simulink model "iso_force_production"  (R2015a)
settings: Solver=ode4  SolverMode=MultiTasking  StartTime=0.0  StopTime=inf  FixedStep=BKIN_STEP_TIME  RelTol=1e-3
StartFcn:
  |  warndlg('Dexterit-E models cannot run under simulation. Please compile your model and run it from within Dexterit-E.');set_param(bdroot,'SimulationCommand','stop')
model workspace (MAT data in the model file):
  BKIN_STEP_TIME = 0.00025
  col_x = 1
  col_y = 2
  VRAD = 3
  COLOR = 4
  TARGET_COL = 1
  BKIN_KINEMATIC_FRAME_SIZE = 400
  E_NO_EVENT = 0
  K_START_TGT = 1
  INIT_DUR = 4
  TP_ITI = 8
  K_JOINT_ASSESSED = 2
  TEXT1 = 5
  TEXT2 = 6
  HEIGHT = 7
  STROKE_WIDTH = 8
  GOAL_F_PCT = 2
  DO_FDBK = 7
  MAX_MOVE_TIME = 6
  FORCE_HOLD_TIME = 5
  MIN_FORCE = 3
  E_TEST_MVC = 1
  E_HOLD_MVC = 3
  E_EOT = 10
  E_FORCE_TRIAL = 2
  E_HOLD_FORCE = 4
libraries: Video x4, General x3, KINARM_loads x2, slrtlib x2, KINARM_IO x1, simulink x1
CloseFcn:
  | rtwprivate ssgencode ModelCloseRequest b2lab2d
settings Model: ModifiedComment=chris -- Wed Feb 16 09:18:30 2005 -- Version 1.1384  ExtModeArmWhenConnect=off  ExtModeLogAll=off  LastModifiedBy=Aaron
settings SolverCC: EnableConcurrentExecution=on  AutoInsertRateTranBlk=on
settings DataIOCC: LimitDataPoints=off  SignalLoggingSaveFormat=ModelDataLogs  SaveOutput=off  SaveTime=off  SignalLoggingName=sigsOut
settings OptimizationCC: BlockReduction=off  BooleanDataType=off  OptimizeBlockIOStorage=off  BufferReuse=off  GlobalBufferReuse=off  ExpressionFolding=off  ExpressionDepthLimit=2147483647  LocalBlockOutputs=off  InitFltsAndDblsToZero=on
settings DebuggingCC: SaveWithParameterizedLinksMsg=none  UnderspecifiedInitializationDetection=Classic  MergeDetectMultiDrivingBlocksExec=none  SignalResolutionControl=TryResolveAllWithWarning  MultiTaskDSMMsg=warning  FcnCallInpInsideContextMsg=UseLocalSettings  StateNameClashWarn=warning  StrictBusMsg=ErrorOnBusTreatedAsVector
settings HardwareCC: ProdIntDivRoundTo=Zero  ProdEndianess=LittleEndian  ProdLongLongMode=on  ProdHWDeviceType=Generic->32-bit x86 compatible  TargetHWDeviceType=32-bit Generic
settings SFSimCC: SimParseCustomCode=off
settings RTWCC: SystemTargetFile=slrt.tlc  TemplateMakefile=slrt_default_tmf  Description=Simulink Real-Time  RTWCompilerOptimization=on
settings CodeAppCC: MaxIdLength=63
settings SimulinkRealTimeCC: TargetFcnLib=ansi_tfl_tmw.mat  GeneratePreprocessorConditionals=Disable all  xPCisDownloadable=off

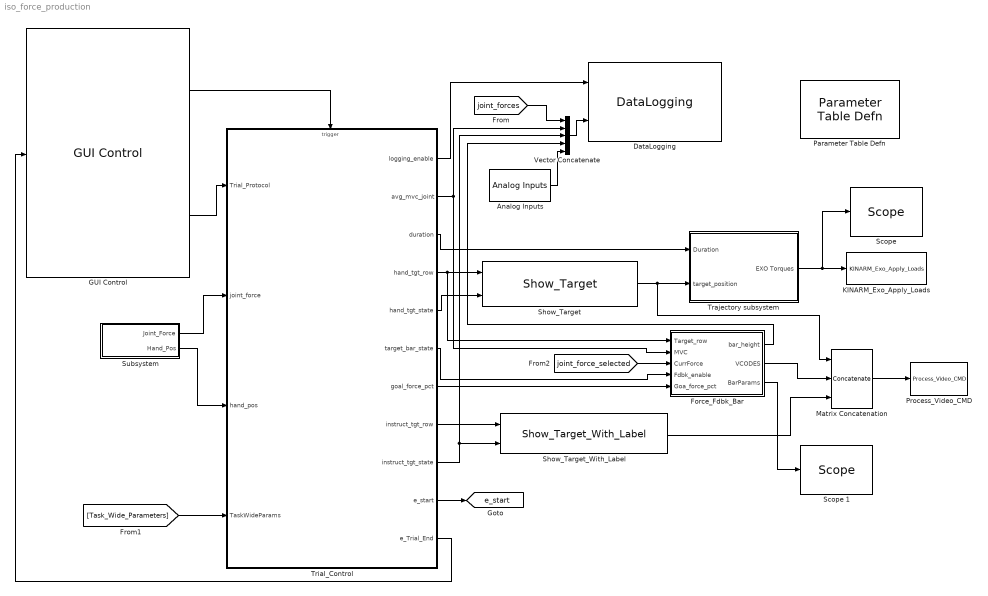
== system iso_force_production ==
  Analog Inputs : KINARM_IO/Analog Inputs  channel=[1]  range=[5]  coupling=[0]  scantime6071e=1.28e-5  scantime6229=5e-6  sampletime=0.001  slot=-1  oscantime6071e=0
  DataLogging : General/DataLogging  log_event_codes=off  log_analog_inputs=on  show_time_remaining=off  ecat_include=on
      link override Poll KINARM/EPTorqueCMD: GotoTag=KINARMEPTorqueCMD
      link override Poll KINARM/TorqueCMD: GotoTag=KINARMTorqueCMD
  Force_Fdbk_Bar : Subsystem
  GUI Control : General/GUI Control  task_version=1.0  show_repeat_trial_flag=off  use_custom_tp=off  target_type_str=Circle  Target_Type=1  XYcols=[1 2]  Vcols=3  Lcols=4  indices_padding=[0 0 0 0;0 0 0 0]  target_table_rows=64  load_table_rows=20  tp_table_rows=100
  KINARM_Exo_Apply_Loads : KINARM_loads/KINARM_Exo_Apply_Loads  up_duration=1000  down_duration=1000  max_torque=1  limit_motors=off
  Matrix Concatenation : Concatenate  NumInputs=3  Mode=Multidimensional array
  Parameter Table Defn : General/Parameter Table Defn  ShowInLibBrowser=0
  Process_Video_CMD : Video/Process_Video_CMD  video_delay=0
  "Scope " : slrtlib/Displays and Logging/Scope   scopeno=1  scopetype=Target  autostart=on  viewmode=Numerical  formatstr='%15.6f'  grid=on  ylimits=[0,0]  nosamples=250  noprepostsamples=0  interleave=1  triggermode=FreeRun  triggersignal=1  trigsignalfromport=off  triggerlevel=0.0  triggerslope=Either  triggerscope=1  triggersample=0  filename=data.dat  mode=Lazy  writesize=512  autorestart=off  dynamicfilemode=off  maxwritefilesize=512*1024^2
  Scope 1 : slrtlib/Displays and Logging/Scope   scopeno=2  scopetype=Target  autostart=on  viewmode=Numerical  formatstr='%15.6f'  grid=on  ylimits=[0,0]  nosamples=250  noprepostsamples=0  interleave=1  triggermode=FreeRun  triggersignal=1  trigsignalfromport=off  triggerlevel=0.0  triggerslope=Either  triggerscope=1  triggersample=0  filename=data.dat  mode=Lazy  writesize=512  autorestart=off  dynamicfilemode=off  maxwritefilesize=512*1024^2
  Show_Target : Video/Show_Target  target_type=Circle  num_states=1  attribcol1=[COLOR 0 0 VRAD]  attribcol2=[0 0 0 0]  attribcol3=[0 0 0 0]  attribcol4=[0 0 0 0]  attribcol5=[0 0 0 0]  stateindices_padding=[0 0 0 0 0 0 0;0 0 0 0 0 0 0;0 0 0 0 0 0 0;0 0 0 0 0 0 0;0 0 0 0 0 0 0]  source=dialog  opacity=100  target_display=Both subject and operator displays  num_col=4
  Show_Target_With_Label : Video/Show_Target_With_Label  target_type=Rectangle  num_states=2  attribcol1=[0 0 0 VRAD HEIGHT 0 TEXT1 COLOR HEIGHT]  attribcol2=[0 0 0 VRAD HEIGHT 0 TEXT2 COLOR HEIGHT]  attribcol3=[0 0 0 0 0 0 0 0 0]  attribcol4=[0 0 0 0 0 0 0 0 0]  attribcol5=[0 0 0 0 0 0 0 0 0]  stateindices_padding=[0 0;0 0;0 0;0 0;0 0]  source=dialog  opacity=100  target_display=Both subject and operator displays
  Subsystem : Subsystem
  Trajectory subsystem : Subsystem
  Trial_Control : Stateflow chart  TreatAsAtomicUnit=on
  Vector Concatenate : Concatenate  NumInputs=5
  tag scope: e_start=global
  wires:
  Show_Target/1 -> Matrix Concatenation/1, Trajectory subsystem/2(target_position)
  Trial_Control/11(e_Trial_End) -> GUI Control/1
  GUI Control/1 -> Trial_Control/Trigger
  Trial_Control/5(hand_tgt_state) -> Show_Target/2
  Trial_Control/4(hand_tgt_row) -> Force_Fdbk_Bar/1(Target_row), Show_Target/1
  Matrix Concatenation/1 -> Process_Video_CMD/1
  GUI Control/2 -> Trial_Control/1(Trial_Protocol)
  Trial_Control/1(logging_enable) -> DataLogging/1
  Trial_Control/3(duration) -> Trajectory subsystem/1(Duration)
  Trajectory subsystem/1(EXO Torques) -> "Scope "/1, KINARM_Exo_Apply_Loads/1
  Trial_Control/10(e_start) -> [e_start]
  [joint_forces] -> Vector Concatenate/1
  Vector Concatenate/1 -> DataLogging/2
  Analog Inputs/1 -> Vector Concatenate/5
  Subsystem/1(Joint_Force) -> Trial_Control/2(joint_force)
  Subsystem/2(Hand_Pos) -> Trial_Control/3(hand_pos)
  [Task_Wide_Parameters] -> Trial_Control/4(TaskWideParams)
  Trial_Control/8(instruct_tgt_row) -> Show_Target_With_Label/1
  Trial_Control/9(instruct_tgt_state) -> Vector Concatenate/3, Show_Target_With_Label/2
  Show_Target_With_Label/1 -> Matrix Concatenation/3
  Trial_Control/2(avg_mvc_joint) -> Force_Fdbk_Bar/2(MVC), Vector Concatenate/2
  Force_Fdbk_Bar/2(VCODES) -> Matrix Concatenation/2
  Trial_Control/6(target_bar_state) -> Force_Fdbk_Bar/4(Fdbk_enable)
  [joint_force_selected] -> Force_Fdbk_Bar/3(CurrForce)
  Trial_Control/7(goal_force_pct) -> Force_Fdbk_Bar/5(Goa_force_pct)
  Force_Fdbk_Bar/1(bar_height) -> Vector Concatenate/4
  Force_Fdbk_Bar/3(BarParams) -> Scope 1/1

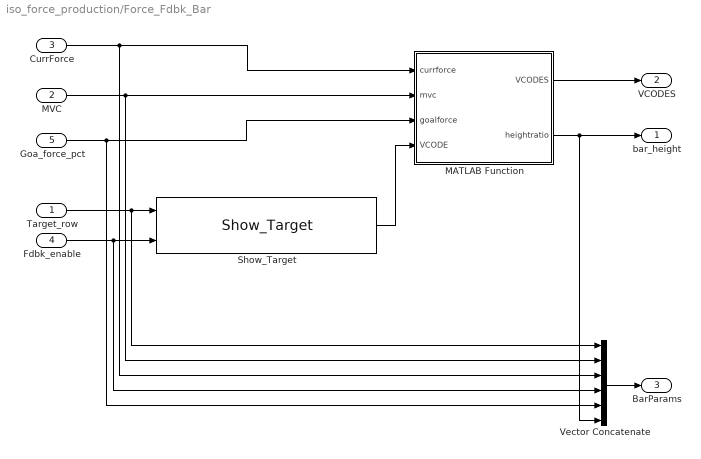
== system iso_force_production/Force_Fdbk_Bar ==
  Target_row : Inport
  MVC : Inport  Port=2
  CurrForce : Inport  Port=3
  Fdbk_enable : Inport  Port=4
  Goa_force_pct : Inport  Port=5
  MATLAB Function : MATLAB Function  TreatAsAtomicUnit=on
  Show_Target : Video/Show_Target  target_type=Rectangle  num_states=1  attribcol1=[COLOR 0 STROKE_WIDTH VRAD HEIGHT 0]  attribcol2=[0 0 0 0 0 0]  attribcol3=[0 0 0 0 0 0]  attribcol4=[0 0 0 0 0 0]  attribcol5=[0 0 0 0 0 0]  stateindices_padding=[0 0 0 0 0;0 0 0 0 0;0 0 0 0 0;0 0 0 0 0;0 0 0 0 0]  source=dialog  opacity=100  target_display=Both subject and operator displays  num_col=6
  Vector Concatenate : Concatenate  NumInputs=6
  bar_height : Outport
  VCODES : Outport  Port=2
  BarParams : Outport  Port=3
  wires:
  Fdbk_enable/1 -> Vector Concatenate/4, Show_Target/2
  Target_row/1 -> Vector Concatenate/1, Show_Target/1
  CurrForce/1 -> Vector Concatenate/3, MATLAB Function/1(currforce)
  MVC/1 -> Vector Concatenate/2, MATLAB Function/2(mvc)
  Show_Target/1 -> MATLAB Function/4(VCODE)
  MATLAB Function/1(VCODES) -> VCODES/1
  Goa_force_pct/1 -> Vector Concatenate/5, MATLAB Function/3(goalforce)
  MATLAB Function/2(heightratio) -> Vector Concatenate/6, bar_height/1
  Vector Concatenate/1 -> BarParams/1

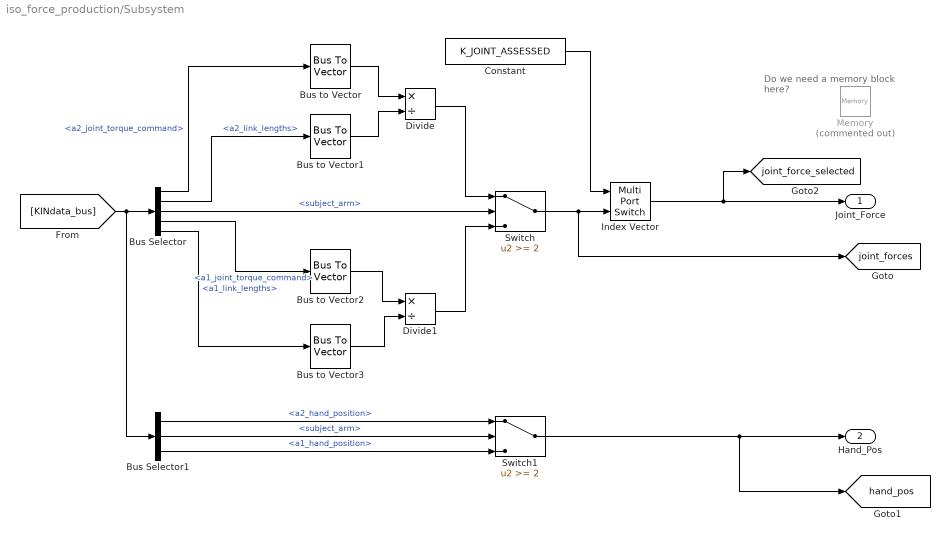
== system iso_force_production/Subsystem ==
  note: Do we need a memory block here?
  Bus Selector : BusSelector  OutputSignals=Robot2.a2_joint_torque_command,Robot2.a2_link_lengths,KINDataGeneral.subject_arm,Robot1.a1_joint_torque_command,Robot1.a1_link_lengths
  Bus Selector1 : BusSelector  OutputSignals=Robot2.a2_hand_position,KINDataGeneral.subject_arm,Robot1.a1_hand_position
  Bus to Vector{,1..3} (4 alike) : BusToVector
  Constant : Constant  Value=K_JOINT_ASSESSED
  Divide : Product  Inputs=*/
  Divide1 : Product  Inputs=*/
  Index Vector : MultiPortSwitch  Inputs=1
  Memory : Memory  Commented=on
  Switch : Switch  Threshold=2
  Switch1 : Switch  Threshold=2
  Joint_Force : Outport
  Hand_Pos : Outport  Port=2
  tag scope: hand_pos=global, joint_force_selected=global, joint_forces=global
  wires:
  [KINdata_bus] -> Bus Selector1/1, Bus Selector/1
  Bus Selector/3 -> Switch/2  "<subject_arm>"
  Bus to Vector/1 -> Divide/1
  Bus to Vector1/1 -> Divide/2
  Bus to Vector2/1 -> Divide1/1
  Bus to Vector3/1 -> Divide1/2
  Divide/1 -> Switch/1
  Divide1/1 -> Switch/3
  Bus Selector/1 -> Bus to Vector/1  "<a2_joint_torque_command>"
  Bus Selector/2 -> Bus to Vector1/1  "<a2_link_lengths>"
  Bus Selector/4 -> Bus to Vector2/1  "<a1_joint_torque_command>"
  Bus Selector/5 -> Bus to Vector3/1  "<a1_link_lengths>"
  Bus Selector1/1 -> Switch1/1  "<a2_hand_position>"
  Bus Selector1/2 -> Switch1/2  "<subject_arm>"
  Bus Selector1/3 -> Switch1/3  "<a1_hand_position>"
  Switch/1 -> [joint_forces], Index Vector/2
  Constant/1 -> Index Vector/1
  Switch1/1 -> [hand_pos], Hand_Pos/1
  Index Vector/1 -> [joint_force_selected], Joint_Force/1

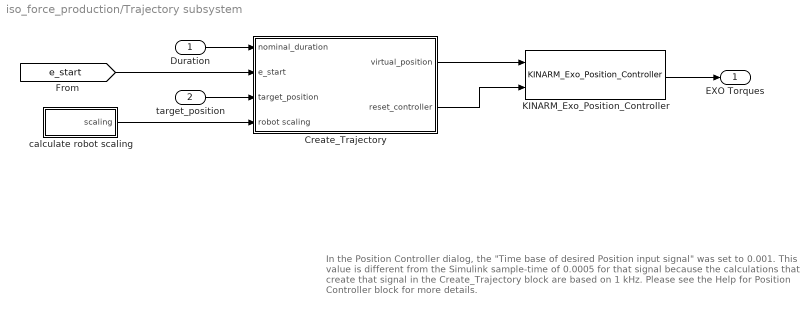
== system iso_force_production/Trajectory subsystem ==
  note: In the Position Controller dialog, the "Time base of desired Position input signal" was set to 0.001.
      | This value is different from the Simulink sample-time of 0.0005 for that signal because the calculations
      | that create that signal in the Create_Trajectory block are based on 1 kHz. Please see the Help for
      | Position Controller block for more details.
  Duration : Inport
  target_position : Inport  Port=2
  Create_Trajectory : Subsystem
  KINARM_Exo_Position_Controller : KINARM_loads/KINARM_Exo_Position_Controller  use_dom_hand=on  KINARM_Type=Human  inertias_for_FF=KINARM robot  angles_or_XY=End-point (global x/y)  sample_time=0.001
  calculate robot scaling : Subsystem
  EXO Torques : Outport
  wires:
  Create_Trajectory/2(reset_controller) -> KINARM_Exo_Position_Controller/2
  Create_Trajectory/1(virtual_position) -> KINARM_Exo_Position_Controller/1
  KINARM_Exo_Position_Controller/1 -> EXO Torques/1
  target_position/1 -> Create_Trajectory/3(target_position)
  Duration/1 -> Create_Trajectory/1(nominal_duration)
  [e_start] -> Create_Trajectory/2(e_start)
  calculate robot scaling/1(scaling) -> Create_Trajectory/4(robot scaling)

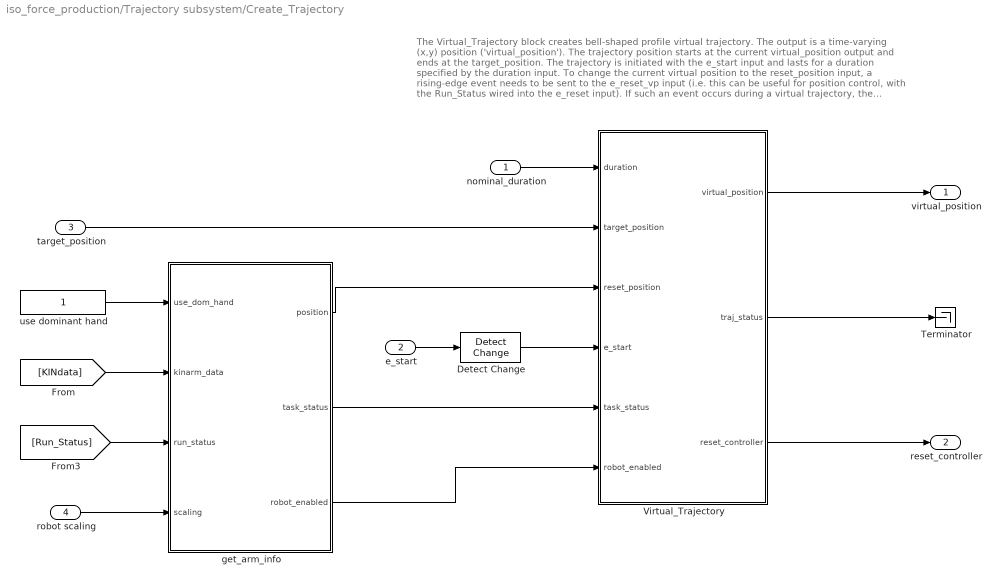
== system iso_force_production/Trajectory subsystem/Create_Trajectory ==
  note: The Virtual_Trajectory block creates bell-shaped profile virtual trajectory.
      | The output is a time-varying (x,y) position ('virtual_position').
      |
      | The trajectory position starts at the current virtual_position output and ends at the target_position.
      | The trajectory is initiated with the e_start input and lasts for a duration specified by the duration input.
      |
      | To change the current virtual position to the reset_position input, a rising-edge event needs to be sent to the e_reset_vp input
      | (i.e. this can be useful for position control, with the Run_Status wired into the e_reset input).
      | If such an event occurs during a virtual trajectory, the trajectory is halted immediately.
  nominal_duration : Inport
  e_start : Inport  Port=2
  target_position : Inport  Port=3
  robot scaling : Inport  Port=4
  Detect Change : simulink/Logic and Bit Operations/Detect Change  vinit=0  InputProcessing=Inherited  OutDataTypeStr=uint8
  Terminator : Terminator
  Virtual_Trajectory : Subsystem
  get_arm_info : MATLAB Function  TreatAsAtomicUnit=on
  use dominant hand : Constant
  virtual_position : Outport
  reset_controller : Outport  Port=2
  wires:
  Virtual_Trajectory/1(virtual_position) -> virtual_position/1
  nominal_duration/1 -> Virtual_Trajectory/1(duration)
  e_start/1 -> Detect Change/1
  target_position/1 -> Virtual_Trajectory/2(target_position)
  Detect Change/1 -> Virtual_Trajectory/4(e_start)
  use dominant hand/1 -> get_arm_info/1(use_dom_hand)
  [KINdata] -> get_arm_info/2(kinarm_data)
  get_arm_info/1(position) -> Virtual_Trajectory/3(reset_position)
  Virtual_Trajectory/3(reset_controller) -> reset_controller/1
  get_arm_info/2(task_status) -> Virtual_Trajectory/5(task_status)
  get_arm_info/3(robot_enabled) -> Virtual_Trajectory/6(robot_enabled)
  [Run_Status] -> get_arm_info/3(run_status)
  Virtual_Trajectory/2(traj_status) -> Terminator/1
  robot scaling/1 -> get_arm_info/4(scaling)

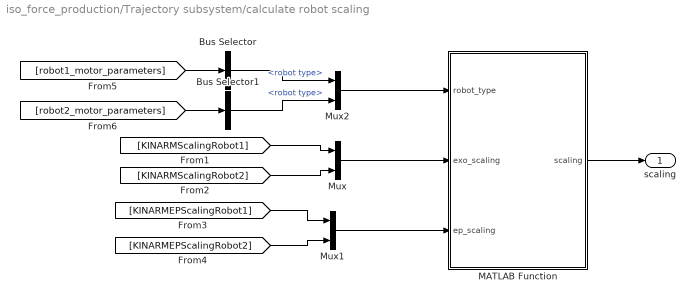
== system iso_force_production/Trajectory subsystem/calculate robot scaling ==
  Bus Selector : BusSelector  OutputSignals=robot type
  Bus Selector1 : BusSelector  OutputSignals=robot type
  MATLAB Function : MATLAB Function  TreatAsAtomicUnit=on
  Mux : Mux  Inputs=2
  Mux1 : Mux  Inputs=2
  Mux2 : Mux  Inputs=2
  scaling : Outport
  wires:
  [KINARMScalingRobot1] -> Mux/1
  [KINARMScalingRobot2] -> Mux/2
  Mux/1 -> MATLAB Function/2(exo_scaling)
  Mux1/1 -> MATLAB Function/3(ep_scaling)
  Mux2/1 -> MATLAB Function/1(robot_type)
  MATLAB Function/1(scaling) -> scaling/1
  [robot2_motor_parameters] -> Bus Selector1/1
  Bus Selector1/1 -> Mux2/2  "<robot type>"
  [KINARMEPScalingRobot2] -> Mux1/2
  [KINARMEPScalingRobot1] -> Mux1/1
  Bus Selector/1 -> Mux2/1  "<robot type>"
  [robot1_motor_parameters] -> Bus Selector/1

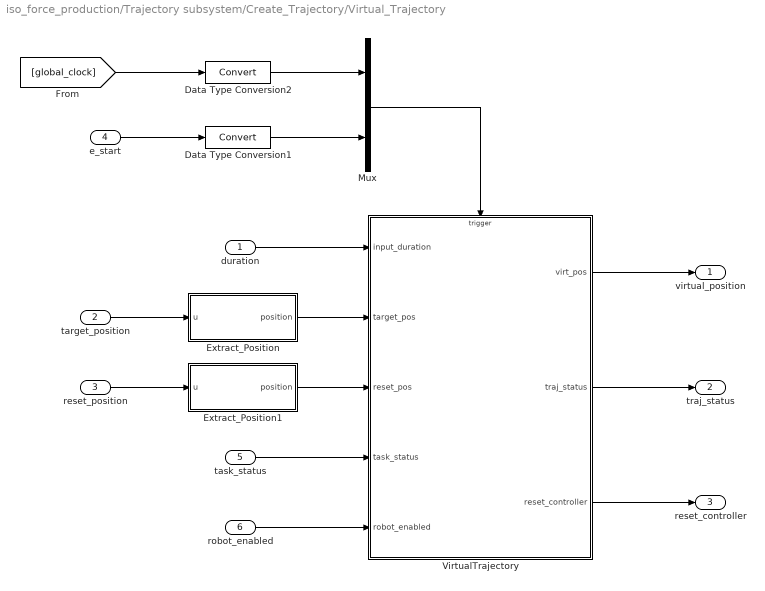
== system iso_force_production/Trajectory subsystem/Create_Trajectory/Virtual_Trajectory ==
  duration : Inport
  target_position : Inport  Port=2
  reset_position : Inport  Port=3
  e_start : Inport  Port=4
  task_status : Inport  Port=5
  robot_enabled : Inport  Port=6
  Data Type Conversion1 : DataTypeConversion
  Data Type Conversion2 : DataTypeConversion
  Extract_Position : MATLAB Function  TreatAsAtomicUnit=on
  Extract_Position1 : MATLAB Function  TreatAsAtomicUnit=on
  Mux : Mux  Inputs=2
  VirtualTrajectory : Stateflow chart  TreatAsAtomicUnit=on
  virtual_position : Outport
  traj_status : Outport  Port=2
  reset_controller : Outport  Port=3
  wires:
  e_start/1 -> Data Type Conversion1/1
  target_position/1 -> Extract_Position/1(u)
  [global_clock] -> Data Type Conversion2/1
  Mux/1 -> VirtualTrajectory/Trigger
  duration/1 -> VirtualTrajectory/1(input_duration)
  VirtualTrajectory/1(virt_pos) -> virtual_position/1
  Extract_Position/1(position) -> VirtualTrajectory/2(target_pos)
  reset_position/1 -> Extract_Position1/1(u)
  Data Type Conversion2/1 -> Mux/1
  VirtualTrajectory/2(traj_status) -> traj_status/1
  robot_enabled/1 -> VirtualTrajectory/5(robot_enabled)
  task_status/1 -> VirtualTrajectory/4(task_status)
  Data Type Conversion1/1 -> Mux/2
  Extract_Position1/1(position) -> VirtualTrajectory/3(reset_pos)
  VirtualTrajectory/3(reset_controller) -> reset_controller/1

== stateflow chart iso_force_production/Trial_Control ==
  settings: sampleTime=0.001
  state init/
    //bring the hand to the start position
    mvc_joint = 0;
    n_mvc = 0;
    avg_mvc_joint = 0;
    hand_tgt_row = TaskWideParams[K_START_TGT];
    hand_tgt_state = 1;
    instruct_tgt_row = 0;
    instruct_tgt_state = 0;
  state MovToStart/
    ITI = Trial_Protocol[TP_ITI];
    MVCtrial = Trial_Protocol[MVC_TRIAL];
    duration = Trial_Protocol[INIT_DUR];
    e_start;
  state Main_Trial
    state InitMVC/
      event_code = E_TEST_MVC;
      logging_enable = 1;
      duration = 1;
      instruct_tgt_row = Trial_Protocol[TARGET_COL];
      instruct_tgt_state = 1;
      tmpforce = 0;
      tmpcounter = 0;
      iforce = 0;
      maxforce = 0;
      min_force = Trial_Protocol[MIN_FORCE];
      force_hold_time = Trial_Protocol[FORCE_HOLD_TIME];
      max_move_time = Trial_Protocol[MAX_MOVE_TIME];
      tick = 0;
    state InitForceTrial/
      event_code = E_FORCE_TRIAL;
      logging_enable = 1;
      duration = 1;
      instruct_tgt_row = Trial_Protocol[TARGET_COL];
      instruct_tgt_state = 1;
      tmpforce = 0;
      tmpcounter = 0;
      iforce = 0;
      maxforce = 0;
      min_force = Trial_Protocol[MIN_FORCE];
      goal_force_pct = Trial_Protocol[GOAL_F_PCT];
      goal_force = avg_mvc_joint*(goal_force*pct)/100.0;
      target_bar_state = Trial_Protocol[DO_FDBK];
      force_hold_time = Trial_Protocol[FORCE_HOLD_TIME];
      max_move_time = Trial_Protocol[MAX_MOVE_TIME];
      tick = 0;
    state MeasureMVC/
      event_code = E_HOLD_MVC;
      during: //check and update the estimated mvc
      [tmpforce, tmpcounter, iforce, maxforce] = update_mvc(tmpforce,joint_force,tmpcounter, iforce, maxforce, min_force);
      tick++;
    state ApplyForce/
      during:
      maxforce = joint_force;
      tmpcounter = 0;
      tick++;
    state EndMVC/
      event_code = E_EOT;
      //record the MVC on this trial if it was a good trial (i.e., it didn't time out)
      mvc_joint += (maxforce)*(tmpcounter >= force_hold_time);
      n_mvc += (1)*(tmpcounter >= force_hold_time);
      avg_mvc_joint = mvc_joint/n_mvc;
      instruct_tgt_state = 2;
    state HoldAppliedForce/
      event_code = E_HOLD_FORCE;
      during:
      maxforce = joint_force;
      tmpcounter++;
      tick++;
    state EndOfTrial/
      event_code = E_EOT;
      instruct_tgt_state = 2;
    InitMVC -> MeasureMVC : [(joint_force > min_force) && after(1, e_clk)]
    InitForceTrial -> ApplyForce : [(joint_force > min_force) && after(1, e_clk)]
    MeasureMVC -> EndMVC : [(tmpcounter >= force_hold_time) || (tick > max_move_time) ]
    ApplyForce -> HoldAppliedForce : [joint_force > goal_force]
    HoldAppliedForce -> ApplyForce [order 1] : [(joint_force - goal_force) <= min_force]
    HoldAppliedForce -> EndOfTrial [order 2] : [(tmpcounter > force_hold_time) || (tick > max_move_time) ]
  state Inter_Trial_State/
    e_Trial_End
  state WaitForFlagToSet
  (default) -> init
  MovToStart -> (junction 75) : after(duration, e_clk)/
      | hand_tgt_state = 0;
  (junction 75) -> InitForceTrial [order 1] : [MVCtrial == 0]/
  (junction 75) -> InitMVC [order 2] : [MVCtrial == 1]
  init -> (junction 85)
  (junction 85) -> MovToStart
  Inter_Trial_State -> (junction 85)
  WaitForFlagToSet -> Inter_Trial_State : after(2, e_clk)
  Main_Trial -> WaitForFlagToSet : e_ExitTrialNow/
      | target_state = 0;
      | logging_enable = 0;
      | tickCount = 10;
  (junction 111) -> Inter_Trial_State : after(ITI, e_clk)
  EndMVC -> (junction 111) : [joint_force <= min_force]
  EndOfTrial -> (junction 111) : [joint_force <= min_force]
  data: currMVC function_input double; currForce function_input double; newMVC function_output double; newcount function_output double; currcount function_input double; imvc function_input double; imvc1 function_output double; max_mvc function_input double; newmax_mvc function_output double; min_force function_input double; logging_enable output boolean; avg_mvc_joint output double; mvc_joint local double; duration output double; hand_tgt_row output [1..32]; hand_tgt_state output double; tickCount local double; Trial_Protocol input double; max_move_time local double size=1; joint_force input double; target_bar_state output double; goal_force_pct output double; hand_pos input double; TaskWideParams input double; instruct_tgt_row output double; instruct_tgt_state output double; n_mvc local double; tmp_force local double size=10; tmp_counter local double; iforce local double; max_force local double; force_hold_time local double
  data hand_tgt_row settings: description=index of the row currently being used in the TargetTable
  events: e_start output EITHER_EDGE_EVENT; e_clk input RISING_EDGE_EVENT; e_ExitTrialNow input EITHER_EDGE_EVENT; e_Trial_End output EITHER_EDGE_EVENT
  function [newMVC,newcount, imvc1, newmax_mvc] = update_mvc(currMVC,currForce, currcount, imvc, max_mvc, min_force):
    | function [newMVC,newcount, imvc1, newmax_mvc] = update_mvc(currMVC,currForce, currcount, imvc, max_mvc, min_force)
    | 
    | meanmvc = mean(currMVC);
    | newMVC = currMVC;
    | 
    | forcethresh = min_force;
    | 
    | %keep a running history of applied forces
    | imvc1 = imvc+1;
    | if imvc1 > length(newMVC)
    |     imvc1 = 1;
    | end
    | 
    | newMVC(imvc1) = currForce;
    | 
    | if (currForce-meanmvc) > forcethresh  %current force is greater than the current average recorded force
    |     newcount = 0;
    |     newmax_mvc = meanmvc;
    | elseif abs(currForce-meanmvc) < forcethresh %current force is within range of current average recorded force
    |     newcount = currcount+1;
    |     newmax_mvc = meanmvc;
    | else %current force is less than range of current average recorded force
    |     currcount = 0;
    |     newmax_mvc = max_mvc;
    | end

== matlab function iso_force_production/Trajectory subsystem/calculate robot scaling/MATLAB Function ==
  data: robot_type input; scaling output; exo_scaling input; ep_scaling input
function scaling = fcn(robot_type, exo_scaling, ep_scaling)
%#codegen

scaling = [0, 0];

%0 = EXO, 1 = EP, 2 = NHP
for n=1:2
    if robot_type(n) == 1
        scaling(n) = ep_scaling(n);
    else
        scaling(n) = exo_scaling(n);
    end
end

== matlab function iso_force_production/Trajectory subsystem/Create_Trajectory/Virtual_Trajectory/Extract_Position ==
  settings: fimath=|
      | fimath(...
      | 'RoundMode', 'floor',...
      | 'OverflowMode', 'wrap',...
      | 'ProductMode', 'KeepLSB', 'ProductWordLength', 32,...
      | 'SumMode', 'KeepLSB', 'SumWordLength', 32,...
      | 'CastBeforeSum', false)
  data: u input; position output
function position = fcn(u)

position=[0,0];	%initialization
if length(u)==2	%input is assumed to be (x,y) position, global coordinates, (m)		
	position=u;
else			%input is assumed to be a VCODE
	position(1)=u(3);
	position(2)=u(4);
end

== matlab function iso_force_production/Trajectory subsystem/Create_Trajectory/Virtual_Trajectory/Extract_Position1 ==
  settings: fimath=|
      | fimath(...
      | 'RoundMode', 'floor',...
      | 'OverflowMode', 'wrap',...
      | 'ProductMode', 'KeepLSB', 'ProductWordLength', 32,...
      | 'SumMode', 'KeepLSB', 'SumWordLength', 32,...
      | 'CastBeforeSum', false)
  data: u input; position output
function position = fcn(u)

position=[0,0];	%initialization
if length(u)==2	%input is assumed to be (x,y) position, global coordinates, (m)		
	position=u;
else			%input is assumed to be a VCODE
	position(1)=u(3);
	position(2)=u(4);
end

== matlab function iso_force_production/Force_Fdbk_Bar/MATLAB Function ==
  data: currforce input; VCODES output; mvc input; goalforce input; VCODE input; heightratio output
function [VCODES,heightratio] = fcn(currforce,mvc,goalforce,VCODE)
%#codegen

%calculate the height ratio to scale the inner bar by
heightratio = currforce/mvc;

%duplicate the rectangle shape; VCODE(1,:) will be the inner fill bar,
% VCODE(2,:) will be the outer border, and VCODE(3,:) will be the goal line
VCODES = [VCODE; VCODE; VCODE];



%VCODE(1,:) specifies a fill color and no stroke color; we want to make the
%outline have no fill and a white border
VCODES(1,7) = 0; %remove the stroke width on the inner bar
VCODES(2,5) = create_color(0,0,0); %set the outer frame fill to black
VCODES(2,6) = create_color(255,255,255); %set the outer frame stroke to white

%the rectangle has dims (10,11,12) = width (x dir), height (y dir), rot
%we want to scale the inner rect height by the heightratio
VCODES(1,11) = VCODES(1,11)*heightratio;
%we need to edit the y position of the inner bar to keep the base fixed at
%the bottom of the outer frame, by subtracting half the height difference
%between the two bars
VCODES(1,4) = VCODES(1,4) - ( VCODES(2,11) - VCODES(1,11) )/2;  



%we need to add in a line representing the target height.
VCODES(3,1) = 4; %set this to be a line segment

frameheight = VCODES(2,11);
framebottom_pos = VCODES(2,4)-(frameheight/2);
goaloffset = frameheight*(goalforce/100);

VCODES(3,4) = framebottom_pos+goaloffset;
VCODES(3,6) = create_color(255,0,0);  %set the goal color to be red

== stateflow chart iso_force_production/Trajectory subsystem/Create_Trajectory/Virtual_Trajectory/VirtualTrajectory ==
  state Initialization/
    virt_pos = reset_pos;
    // this initialization ensures that the virtual position
    // starts off as something reasonable
    traj_status = 0;   // initialize trajectory status
  state main/
    state wait_for_trigger/
      reset_controller = 0;
    state wait_1_ms_b/
      // wait for controller
      // to be reset
    state on_ramp/
      entry: tick = 0;    // initialize the tick counter
      reset_controller = 0;
      final_pos = target_pos;   // set the final position of the trajectory
      start_pos = virt_pos;   // set the start position of the trajectory
      duration = input_duration;   // store the duration of the trajectory
      traj_status = 1;   // indicate an ongoing trajectory
      during:
      on e_clk: tick++;
      // the trajectory velocity will have a bell shaped profile
      trajectory_shape = tick/duration-sin(2*pi*tick/duration)/(2*pi);
      virt_pos[1] = start_pos[1] + (final_pos[1] - start_pos[1]) * trajectory_shape;
      virt_pos[2] = start_pos[2] + (final_pos[2] - start_pos[2]) * trajectory_shape;
    main -> wait_1_ms_b [order 1] : [(robot_enabled == 1) && (traj_status == -1)]/
        | traj_status = 1;
        | virt_pos = reset_pos;
        | reset_controller = 1;
        | // trajectory was halted and
        | //is now being re-started
    wait_for_trigger -> (junction 20) : e_start
    (junction 20) -> wait_for_trigger [order 2]
    wait_1_ms_b -> (junction 20) : after(1, e_clk)
    (junction 20) -> on_ramp [order 1] : [input_duration>0]
    on_ramp -> wait_for_trigger [order 2] : [robot_enabled == 0]/
        | traj_status = -1;
        | // robot disabled
    on_ramp -> wait_for_trigger [order 1] : after(duration, e_clk)/
        | traj_status = 0
        | // trajectory completed
  state wait_1_ms/
    // wait for controller
    // to be reset
  state task_not_running/
    // wait for task_status to change
    // keep updating virt_pos so that the feedback
    // controller output, which is filtered, does not become
    // huge, resulting in a 'bump' if we don't do this.
    traj_status = 0;
    reset_controller = 0;
    during:
    virt_pos = reset_pos;
  (default) -> Initialization
  Initialization -> wait_for_trigger
  wait_1_ms -> wait_for_trigger : after(1, e_clk)
  task_not_running -> wait_1_ms : [task_status > 0]/
      | reset_controller = 1;
      | // task is running again,
      | // so reset position controller
  main -> task_not_running [order 1] : [task_status == 0]/
      | // means that run_status == 0
      | // AND that torque scaling at
      | // end of task is finished
  data: input_duration input double; target_pos input double size=[1 2]; tick local double; duration local double; reset_pos input double size=[1 2]; task_status input double; pi constant double =3.14159265358979; trajectory_shape local double; virt_pos output double size=[1 2]; traj_status output double; robot_enabled input double; start_pos local double size=[1 2]; final_pos local double size=[1 2]; reset_controller output double
  events: e_clk input RISING_EDGE_EVENT; e_start input RISING_EDGE_EVENT

== matlab function iso_force_production/Trajectory subsystem/Create_Trajectory/get_arm_info ==
  settings: fimath=|
      | fimath(...
      | 'RoundMode', 'floor',...
      | 'OverflowMode', 'wrap',...
      | 'ProductMode', 'KeepLSB', 'ProductWordLength', 32,...
      | 'SumMode', 'KeepLSB', 'SumWordLength', 32,...
      | 'CastBeforeSum', false)
  data: position output; task_status output; use_dom_hand input; kinarm_data input; run_status input; scaling input; robot_enabled output
function [position, task_status, robot_enabled]  = fcn(use_dom_hand, kinarm_data, run_status, scaling)
%
% get current hand position and robot enabled status
%
% May 2009
%

hpx_index = 23;
hpy_index = 24;
robot_disabled_index = 37;

%determine which arm to apply the load to
dominant_hand=kinarm_data(3,1);						%kinarm_data(3,1) tells which arm is the dominant arm
if use_dom_hand == 1
	feedback_arm = dominant_hand;
else
	feedback_arm = 3 - dominant_hand;
end

hpx = kinarm_data( feedback_arm, hpx_index );
hpy = kinarm_data( feedback_arm, hpy_index );
position = [hpx hpy];

if kinarm_data( feedback_arm, robot_disabled_index ) == 0;
    robot_enabled = 1;
else
    robot_enabled = 0;
end

% if the task has stopped/paused (i.e. run_status == 0) AND the torques outputs
% have scaled down to 0, then set the task_status = 0.
if run_status == 0 && scaling(feedback_arm) == 0
    task_status = 0;
else
    task_status = 1;
end
